simulink subsystem "finModel"  (R2026a)
settings: Solver=VariableStepAuto
model mask{finAngles_rad=[0, 0, 0], finCP_m=[0,0,0]}
  mask prompts: finAngles_rad "Fin angle (roll, pitch, yaw) (rad)"; finCP_m "Fin CP location (m)"
values from neighbouring files (symbols this model uses):
  aeroParams : value not decoded    [plantParams.sldd]
  vehicleParams = 18.0    [plantParams.sldd]
libraries: matrix_library x2, aerolibutil x2, simulink_extras x1
settings Model: DataDictionary=plantParams.sldd  EnableAccessToBaseWorkspace=off  Creator=maxhu  LastModifiedBy=maxhu

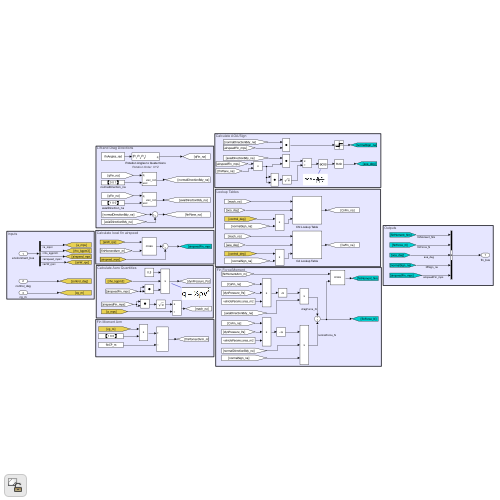
[thumbnail: Simulink's stored preview of the top-level diagram]
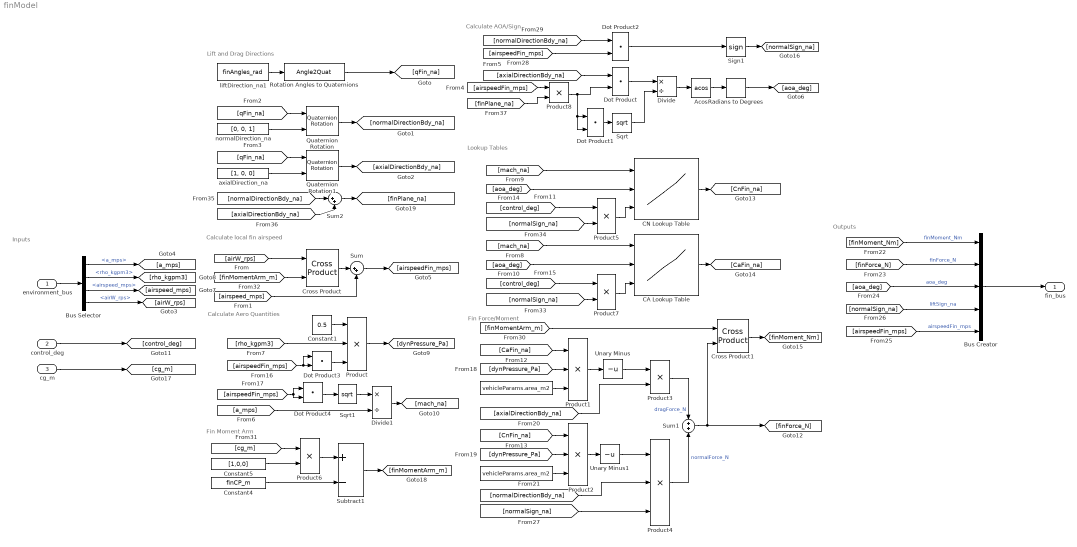
== system finModel ==
  note: Fin Moment Arm
  note: Outputs
  note: Fin Force/Moment
  note: Inputs
  note: Calculate Aero Quantities
  note: Calculate AOA/Sign
  note: Calculate local fin airspeed
  note: Lift and Drag Directions
  note: Lookup Tables
  environment_bus : Inport
  control_deg : Inport  Port=2
  cg_m : Inport  Port=3
  " " : Constant  Value=vehicleParams.area_m2
  "   " : Constant  Value=vehicleParams.area_m2
  Acos : Trigonometry  Operator=acos
  Bus Creator : BusCreator  Inputs=5
  Bus Selector : BusSelector  OutputSignals=a_mps,rho_kgpm3,airspeed_mps,airW_rps
  CA Lookup Table : Lookup_n-D  NumberOfTableDimensions=3  BreakpointsForDimension1=aeroParams.machBreakpoints_na  BreakpointsForDimension2=aeroParams.aoaBreakpoints_deg  BreakpointsForDimension3=aeroParams.controlBreakpoints_deg  Table=aeroParams.CaFin_na  InternalRulePriority=Speed  RndMeth=Simplest
      settings: InputPortMap=u0,u1,u2
  CN Lookup Table : Lookup_n-D  NumberOfTableDimensions=3  BreakpointsForDimension1=aeroParams.machBreakpoints_na  BreakpointsForDimension2=aeroParams.aoaBreakpoints_deg  BreakpointsForDimension3=aeroParams.controlBreakpoints_deg  Table=aeroParams.CnFin_na  InternalRulePriority=Speed  RndMeth=Simplest
      settings: InputPortMap=u0,u1,u2
  Constant1 : Constant  Value=0.5
  Constant4 : Constant  Value=finCP_m
  Constant5 : Constant  Value=[1,0,0]
  Cross Product : matrix_library/Cross Product
  Cross Product1 : matrix_library/Cross Product
  Divide : Product  Inputs=*/
  Divide1 : Product  Inputs=*/
  Dot Product{,1..4} (5 alike) : DotProduct  OutDataTypeStr=Inherit: Inherit via internal rule
  Product{,1..2,4} (4 alike) : Product  Inputs=3
  Product{3,5..8} (5 alike) : Product
  Quaternion Rotation : aerolibutil/Quaternion Rotation
  Quaternion Rotation1 : aerolibutil/Quaternion Rotation
  Radians to Degrees : simulink_extras/Transformations/Radians to Degrees
  Rotation Angles to Quaternions : Angle2Quat  rotationOrder=XYZ
      settings: AttributesFormatString=Rotation Order: %<rotationOrder>
  Sign1 : Signum
  Sqrt : Sqrt
  Sqrt1 : Sqrt
  Subtract1 : Sum  Inputs=+-
  Sum : Sum  Inputs=|++
  Sum1 : Sum  Inputs=+|+
  Sum2 : Sum  Inputs=|++
  Unary Minus : UnaryMinus
  Unary Minus1 : UnaryMinus
  axialDirection_na : Constant  Value=[1, 0, 0]
  liftDirection_na1 : Constant  Value=finAngles_rad
  normalDirection_na : Constant  Value=[0, 0, 1]
  fin_bus : Outport
  wires:
  Sum/1 -> [airspeedFin_mps]
  Cross Product/1 -> Sum/1
  [airspeed_mps] -> Sum/2
  liftDirection_na1/1 -> Rotation Angles to Quaternions/1
  Rotation Angles to Quaternions/1 -> [qFin_na]
  [qFin_na] -> Quaternion Rotation/1
  normalDirection_na/1 -> Quaternion Rotation/2
  [qFin_na] -> Quaternion Rotation1/1
  axialDirection_na/1 -> Quaternion Rotation1/2
  Quaternion Rotation/1 -> [normalDirectionBdy_na]
  Quaternion Rotation1/1 -> [axialDirectionBdy_na]
  [axialDirectionBdy_na] -> Dot Product/1
  Dot Product1/1 -> Sqrt/1
  Dot Product/1 -> Divide/1
  Sqrt/1 -> Divide/2
  Divide/1 -> Acos/1
  Acos/1 -> Radians to Degrees/1
  Radians to Degrees/1 -> [aoa_deg]
  [aoa_deg] -> CN Lookup Table/2
  CN Lookup Table/1 -> [CnFin_na]
  environment_bus/1 -> Bus Selector/1
  Bus Selector/3 -> [airspeed_mps]  "<airspeed_mps>"
  Bus Selector/2 -> [rho_kgpm3]  "<rho_kgpm3>"
  Bus Selector/1 -> [a_mps]  "<a_mps>"
  Product/1 -> [dynPressure_Pa]
  Constant1/1 -> Product/1
  [rho_kgpm3] -> Product/2
  [airspeedFin_mps] -> Dot Product3/2, Dot Product3/1
  Dot Product3/1 -> Product/3
  [a_mps] -> Divide1/2
  Divide1/1 -> [mach_na]
  [mach_na] -> CN Lookup Table/1
  control_deg/1 -> [control_deg]
  [dynPressure_Pa] -> Product1/2
  Product1/1 -> Unary Minus/1
  [CaFin_na] -> Product1/1
  "   "/1 -> Product1/3
  Unary Minus/1 -> Product3/1
  [axialDirectionBdy_na] -> Product3/2
  Product3/1 -> Sum1/1  "dragForce_N"
  [CnFin_na] -> Product2/1
  [normalDirectionBdy_na] -> Product4/2
  Product2/1 -> Unary Minus1/1
  Unary Minus1/1 -> Product4/1
  " "/1 -> Product2/3
  [dynPressure_Pa] -> Product2/2
  Product4/1 -> Sum1/2  "normalForce_N"
  Sum1/1 -> [finForce_N], Cross Product1/2
  Cross Product1/1 -> [finMoment_Nm]
  [aoa_deg] -> Bus Creator/3  "aoa_deg"
  [finForce_N] -> Bus Creator/2  "finForce_N"
  [finMoment_Nm] -> Bus Creator/1  "finMoment_Nm"
  Bus Creator/1 -> fin_bus/1
  Sign1/1 -> [normalSign_na]
  [airspeedFin_mps] -> Bus Creator/5  "airspeedFin_mps"
  [normalSign_na] -> Bus Creator/4  "liftSign_na"
  [normalSign_na] -> Product4/3
  [airspeedFin_mps] -> Dot Product2/2
  [normalDirectionBdy_na] -> Dot Product2/1
  Dot Product2/1 -> Sign1/1
  Sqrt1/1 -> Divide1/1
  [finMomentArm_m] -> Cross Product/2
  [airW_rps] -> Cross Product/1
  Bus Selector/4 -> [airW_rps]  "<airW_rps>"
  cg_m/1 -> [cg_m]
  [cg_m] -> Product6/1
  Product6/1 -> Subtract1/1
  Subtract1/1 -> [finMomentArm_m]
  Constant5/1 -> Product6/2
  Constant4/1 -> Subtract1/2
  [finMomentArm_m] -> Cross Product1/1
  Dot Product4/1 -> Sqrt1/1
  [airspeedFin_mps] -> Dot Product4/2, Dot Product4/1
  Product5/1 -> CN Lookup Table/3
  [normalSign_na] -> Product5/2
  [control_deg] -> Product5/1
  [aoa_deg] -> CA Lookup Table/2
  [normalSign_na] -> Product7/2
  [mach_na] -> CA Lookup Table/1
  Product7/1 -> CA Lookup Table/3
  CA Lookup Table/1 -> [CaFin_na]
  [control_deg] -> Product7/1
  [airspeedFin_mps] -> Product8/1
  Product8/1 -> Dot Product1/1, Dot Product1/2, Dot Product/2
  [normalDirectionBdy_na] -> Sum2/1
  [axialDirectionBdy_na] -> Sum2/2
  Sum2/1 -> [finPlane_na]
  [finPlane_na] -> Product8/2
